simulink model "momentumBasedFlying"  (Simulink 10.2)
settings: Solver=FixedStepAuto  StartTime=0.0  StopTime=Config.simulationTime  FixedStep=Config.tStep  RelTol=1e-3
InitFcn:
  | cd(fileparts(which(bdroot)));
  | initMomentumBasedFlying;
StopFcn:
  | cd(fileparts(which(bdroot)));
  | stopMomentumBasedFlying;
undefined symbols (not defined in the file or in its folder): biasVectorConstraint_feet, Config, confVisualizer, ConstraintMatrix_feet, DiscIntNeverNeededParam, jets_config
libraries: WBToolboxLibrary x86
(part 4 of 4)

== matlab function FLYING CONTROLLER (CORE) V2.5/Flying Controller v2.5/Momentum Control for Flying/extendedKalmanFilter4jets/EKF_jet1/EKF  ==
  data: x input double; input input double; measurement input double; xDot output double; P input double; Config parameter double; Pdot output double
function [xDot, Pdot] = extendedKalmanFilterFNC(x, input, measurement, P, Config)

[xDot, Pdot] = extKalmanFilter(x, input, Config.jetC_P100, P, measurement, Config);

== matlab function FLYING CONTROLLER (CORE) V2.5/Flying Controller v2.5/Momentum Control for Flying/extendedKalmanFilter4jets/EKF_jet1/splitVector ==
  data: x input double; x1 output double; x2 output double
function [x1, x2] = fcn(x)
x1 = x(1);
x2 = x(2);

== matlab function iRonCub/Forward Dynamics/old_simulator_subsystem/Compute generalized external wrench and jet thrust/Compute generalized jet wrench/Jet Dynamics ==
  data: u input double; jetDerivativesOut output double; jetIntensities input double size=[4,1]; jetDerivatives input double size=[4,1]; Config parameter double; jetAccelerationOut output double
function [jetDerivativesOut, jetAccelerationOut] = fcn(u, jetIntensities, jetDerivatives, Config)
jetDerivativesOut = zeros(4,1);
jetAccelerationOut = zeros(4,1);
for i=1:4
    state = [jetIntensities(i), jetDerivatives(i)];
    x = jetModel.get_xDot(state, Config.jet.coeff(i,:), u(i));
    jetDerivativesOut(i) = x(1);
    jetAccelerationOut(i) = x(2);
end
end

== matlab function FLYING CONTROLLER (CORE) V2.5/Flying State Machine/Compute Gains And References/Trajectory Generator/Compute CoM and Base Rotation References ==
  data: posCoM_init input double; w_R_b_init input double; moveFront input double; pos_vel_acc_jerk_CoM_des output double; moveLateral input double; moveUpDown input double; rotateRoll input double; rotatePitch input double; rotateYaw input double; turbo_mode input double; goLandingPos input double; feetContactIsActive input double; oneFootIsInContact input double; t input double; Config parameter double; rot_vel_acc_jerk_base_des output double
function [pos_vel_acc_jerk_CoM_des, rot_vel_acc_jerk_base_des] = ...
             computeReferencesBaseAndCoMFCN(posCoM_init, w_R_b_init, moveFront, moveLateral, moveUpDown, rotateRoll, rotatePitch, ...
                                            rotateYaw, turbo_mode, goLandingPos, feetContactIsActive, oneFootIsInContact, t, Config)
                                     
    [pos_vel_acc_jerk_CoM_des, rot_vel_acc_jerk_base_des] = ...
        computeReferencesBaseAndCoM(posCoM_init, w_R_b_init, moveFront, moveLateral, moveUpDown, rotateRoll, rotatePitch, ...
                                    rotateYaw, turbo_mode, goLandingPos, feetContactIsActive, oneFootIsInContact, t, Config);
end

== matlab function FLYING CONTROLLER (CORE) V2.5/Flying State Machine/Compute Gains And References/Trajectory Generator/Detect Robot Movement Request From Joystick ==
  data: joyAxes input double; moveFront output double; moveLateral output double; moveUpDown output double; rotateRoll output double; rotatePitch output double; joyButtons input double; rotateYaw output double; turbo_mode output double; goLandingPos output double
function [moveFront, moveLateral, moveUpDown, rotateRoll, rotatePitch, rotateYaw, turbo_mode, goLandingPos] = detectMovementsFromJoystickFCN(joyAxes,joyButtons)

    [moveFront, moveLateral, moveUpDown, rotateRoll, rotatePitch, rotateYaw, turbo_mode, goLandingPos] = detectMovementsFromJoystick(joyAxes,joyButtons);
end

== matlab function iRonCub/Forward Dynamics/old_simulator_subsystem/Dynamics and Kinematics/Kinematic Quantities/Compute Thrusts Axes and Arms/Thrust Axes and Arms ==
  data: w_H_J1 input double; matrixOfJetsAxes output double; w_H_J2 input double; w_H_J3 input double; w_H_J4 input double; posCoM input double; matrixOfJetsArms output double; Config parameter double
function [matrixOfJetsAxes, matrixOfJetsArms] = computeJetsAxesAndArmsFCN(w_H_J1, w_H_J2, w_H_J3, w_H_J4, posCoM, Config)

    [matrixOfJetsAxes, matrixOfJetsArms] = computeJetsAxesAndArms(w_H_J1, w_H_J2, w_H_J3, w_H_J4, posCoM, Config);
end

== matlab function FLYING CONTROLLER (CORE) V2.5/Flying State Machine/Compute Gains And References/Smooth CoM and Base References/Smooth Reference Orientations/Rotational PID Controller/Compute Rotation Matrix Derivative ==
  data: gainSmoothingBaseRot input double; w_R_b_des input double; w_R_b input double; b_omega_b output double; RDot output double
function [b_omega_b, RDot] = rotationDerivativeFromAngVelFCN(gainSmoothingBaseRot, w_R_b_des, w_R_b)
                                                                                                                                                            
    % Rotational PID: 
    %
    % w_R_b_des = reference rotation (may be discontinuous)
    % 
    % b_omega_b = control input for the rotational PID. The angular velocity
    %             is expressed w.r.t. a frame attached to the link, i.e. it 
    %             is expressed in the "body" frame (b).
    % 
    % Kp        = control gain
    %
    % w_R_b     = smooth base rotation
    %
    b_omega_b_des       = zeros(3,1);
    Kp                  = gainSmoothingBaseRot;
    b_omega_b           = rotationalPID_bodyVelocity(w_R_b, w_R_b_des, b_omega_b_des, Kp);
                      
    % compute the rotation matrix derivative given the angular velocity in body frame
    RDot                = rotationDerivativeFromBodyAngVel(b_omega_b, w_R_b); 
end

== matlab function iRonCub/Forward Dynamics/old_simulator_subsystem/Compute generalized external wrench and jet thrust/Compute generalized jet wrench/compute_jet_wrenches  ==
  data: matrix_of_jet_axis input double; wrenches_vector output double; jet_intensities input double
function wrenches_vector = compute_jet_wrenches(matrix_of_jet_axis, jet_intensities)
dim_wrench = 6;
num_jets = 4;

% the jets produce pure force (no momentum)
% the wrench is a 6dim vector [Fx, Fy, Fz, 0, 0, 0].transpose

wrenches_vector = zeros(dim_wrench*num_jets, 1);
for i=0:(num_jets-1)
    wrenches_vector(dim_wrench*i + 1: dim_wrench*i + dim_wrench/2) = matrix_of_jet_axis(:,i+1)*jet_intensities(i+1);
end

== matlab function iRonCub/Forward Dynamics/old_simulator_subsystem/State Integration/get_R_dot  ==
  data: R input double size=[3, 3]; omega input double size=[3, 1]; dot_R output double size=[3, 3]
function dot_R = get_R_dot(R, omega)
    dot_R = get_R_dot(R, omega);
end

== matlab function iRonCub/Forward Dynamics/old_simulator_subsystem/State Integration/Homogeneous_matrix  ==
  data: p input double; H output double; R input double
function H = Rp2Hom(p, R)
    H = Rp2Hom(R, p);
end

== matlab function FLYING CONTROLLER (CORE) V2.5/Flying Controller v2.5/Momentum Control for Flying/Feedback linearization/MATLAB Function ==
  data: jets input double; jets_dot input double; jets_dot_des input double; throttle output double size=[4,1]; Config parameter double; error output double; integral_err input double
function [throttle, error]  = fl_jet_control(jets, jets_dot, jets_dot_des, Config, integral_err)

[throttle, error]  = fl_jet_control(jets, jets_dot, jets_dot_des, Config, integral_err);
end

== matlab function FLYING CONTROLLER (CORE) V2.5/Flying Controller v2.5/Momentum Control for Flying/extendedKalmanFilter4jets/EKF_jet2/EKF  ==
  data: x input double; input input double; measurement input double; xDot output double; P input double; Config parameter double; Pdot output double
function [xDot, Pdot] = extendedKalmanFilterFNC(x, input, measurement, P, Config)

[xDot, Pdot] = extKalmanFilter(x, input, Config.jetC_P100, P, measurement, Config);

== matlab function FLYING CONTROLLER (CORE) V2.5/Flying Controller v2.5/Momentum Control for Flying/extendedKalmanFilter4jets/EKF_jet2/splitVector ==
  data: x input double; x1 output double; x2 output double
function [x1, x2] = fcn(x)
x1 = x(1);
x2 = x(2);

== matlab function FLYING CONTROLLER (CORE) V2.5/Flying Controller v2.5/Momentum Control for Flying/extendedKalmanFilter4jets/EKF_jet3/EKF  ==
  data: x input double; input input double; measurement input double; xDot output double; P input double; Config parameter double; Pdot output double
function [xDot, Pdot] = extendedKalmanFilterFNC(x, input, measurement, P, Config)

[xDot, Pdot] = extKalmanFilter(x, input, Config.jetC_P220, P, measurement, Config);

== matlab function FLYING CONTROLLER (CORE) V2.5/Flying Controller v2.5/Momentum Control for Flying/extendedKalmanFilter4jets/EKF_jet3/splitVector ==
  data: x input double; x1 output double; x2 output double
function [x1, x2] = fcn(x)
x1 = x(1);
x2 = x(2);

== matlab function FLYING CONTROLLER (CORE) V2.5/Flying Controller v2.5/Momentum Control for Flying/extendedKalmanFilter4jets/EKF_jet4/EKF  ==
  data: x input double; input input double; measurement input double; xDot output double; P input double; Config parameter double; Pdot output double
function [xDot, Pdot] = extendedKalmanFilterFNC(x, input, measurement, P, Config)

[xDot, Pdot] = extKalmanFilter(x, input, Config.jetC_P220, P, measurement, Config);

== matlab function FLYING CONTROLLER (CORE) V2.5/Flying Controller v2.5/Momentum Control for Flying/extendedKalmanFilter4jets/EKF_jet4/splitVector ==
  data: x input double; x1 output double; x2 output double
function [x1, x2] = fcn(x)
x1 = x(1);
x2 = x(2);
